simulink model "ISA"  (R2018b)
settings: Solver=FixedStepDiscrete  StartTime=0.0  StopTime=10  FixedStep=0.01  RelTol=1e-3
PreLoadFcn:
  | librarySetup
  | eval([bdroot,'_startup']) %Calling [modelName]_startup.m
values from neighbouring files (symbols this model uses):
  PWM_motor = 0.6    [ISA_simulation_startup.m]    (also in ISA_startup.m)
  V_max = 50    [ISA_startup.m]
libraries: HANcoder_STM32_Target x5, HANcoder_STM32_Target2009b x2, simulink x1
CloseFcn:
  | rtwprivate ssgencode ModelCloseRequest mytest
settings Model: Creator=Saliou  LastModifiedBy=Saliou
settings SolverCC: PositivePriorityOrder=on
settings DataIOCC: LimitDataPoints=on  SaveFormat=Array  SaveOutput=off  SaveTime=off
settings OptimizationCC: BlockReduction=off  DefaultParameterBehavior=Inlined  DefaultUnderspecifiedDataType=single  InlineInvariantSignals=on  ExpressionDepthLimit=2147483647  StateBitsets=on  DataBitsets=on  ZeroExternalMemoryAtStartup=off  ZeroInternalMemoryAtStartup=off  InitFltsAndDblsToZero=on  NoFixptDivByZeroProtection=on  EfficientFloat2IntCast=on  LifeSpan=inf
settings DebuggingCC: SaveWithDisabledLinksMsg=none  SaveWithParameterizedLinksMsg=none  CheckSSInitialOutputMsg=off  UnderspecifiedInitializationDetection=Classic  MergeDetectMultiDrivingBlocksExec=none  SignalResolutionControl=TryResolveAll  SolverPrmCheckMsg=warning  InheritedTsInSrcMsg=none  MultiTaskDSMMsg=warning  MultiTaskCondExecSysMsg=none  ParameterPrecisionLossMsg=none  FcnCallInpInsideContextMsg=warning  StateNameClashWarn=warning  SFUnexpectedBacktrackingDiag=warning  SFNoUnconditionalDefaultTransitionDiag=warning  SFExecutionAtInitializationDiag=none
settings HardwareCC: ProdBitPerPointer=32  ProdBitPerSizeT=32  ProdBitPerPtrDiffT=32  ProdLargestAtomicInteger=Long  ProdLargestAtomicFloat=Double  ProdWordSize=32  ProdHWDeviceType=ARM Compatible->ARM Cortex  TargetEndianess=LittleEndian  TargetHWDeviceType=Infineon->TriCore
settings ModelReferenceCC: PropagateSignalLabelsOutOfModel=off
settings SFSimCC: SimUseLocalCustomCode=off  MATLABDynamicMemAlloc=off
settings RTWCC: SystemTargetFile=ert.tlc  MakeCommand=make_rtw SHELL= HANcoder_PORTABLE=1 HANcoder_BOOTLOADER=1  TemplateMakefile=Olimexino_STM32_gcc.tmf  Description=Real-Time Workshop Embedded Coder (no auto configuration)  RTWUseLocalCustomCode=off
settings CodeAppCC: ForceParamTrailComments=on  IgnoreCustomStorageClasses=off  SimulinkDataObjDesc=on  CustomSymbolStrGlobalVar=rt$N$M  CustomSymbolStrType=$N$M  CustomSymbolStrFcn=$N$M$F  CustomSymbolStrMacro=$N$M  InsertBlockDesc=on  StateflowObjectComments=on  InternalIdentifier=Classic
settings ERTTargetCC: TargetFcnLib=ansi_tfl_tmw.mat  MultiwordLength=2048  IncludeMdlTerminateFcn=off  SuppressErrorStatus=on  SupportNonFinite=off  GenerateASAP2=on  InlinedParameterPlacement=NonHierarchical  ERTCustomFileTemplate=example_file_process.tlc  ConvertIfToSwitch=off  SuppressUnreachableDefaultCases=off
settings ConfigComp: CovMetricSettings=dw  CovHtmlReporting=on  CovSaveCumulativeToWorkspaceVar=on  CovSaveSingleToWorkspaceVar=on  CovExternalEMLEnable=off  CovSFcnEnable=off  DVMaxProcessTime=600  DVDisplayUnsatisfiableObjectives=on  DVAutomaticStubbing=off  DVModelCoverageObjectives=MCDC  DVMaxTestCaseSteps=500  DVTestSuiteOptimization=CombinedObjectives  DVDetectActiveLogic=on  DVSaveHarnessModel=on

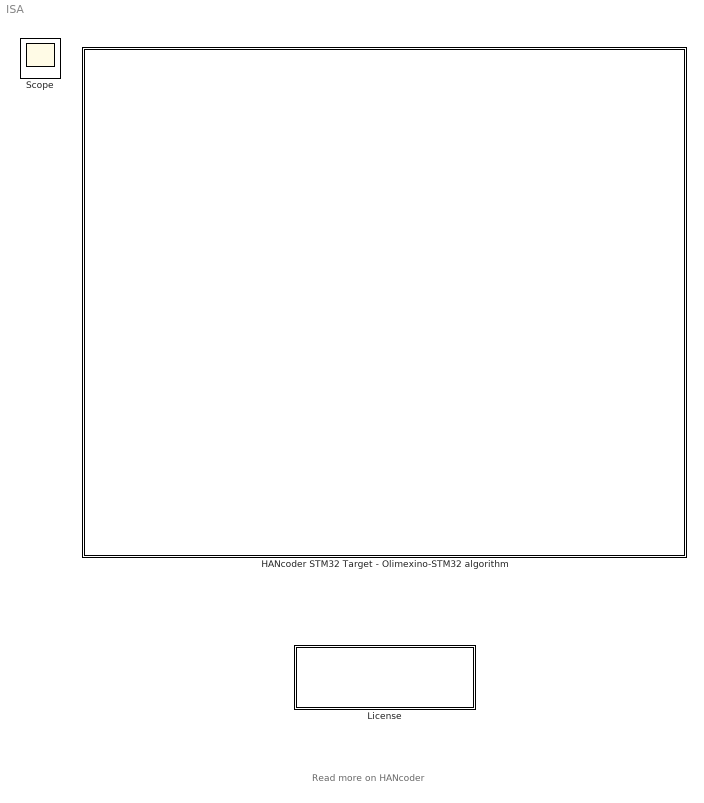
== system ISA ==
  note: Read more on HANcoder
  HANcoder STM32 Target - Olimexino-STM32 algorithm : Subsystem  mask(TopLevelSubsystem){}
      settings: CopyFcn=HANcoderChecks('Copy');  NameChangeFcn=HANcoderChecks('NameChangeOlimexino');  MoveFcn=HANcoderChecks('MoveOlimexino');
      mask Display: image(imread('Olimexino_STM32_HAN.jpg'))
  License : Subsystem  mask(License){}
      settings: NameChangeFcn=HANcoderChecks('NameChangeLicenseBlock');  OpenFcn=winopen('License.pdf')  MoveFcn=HANcoderChecks('MoveLicenseBlock');
      mask Display: disp(['End-User License Agreement\n','please read before use']);
  Scope : Scope

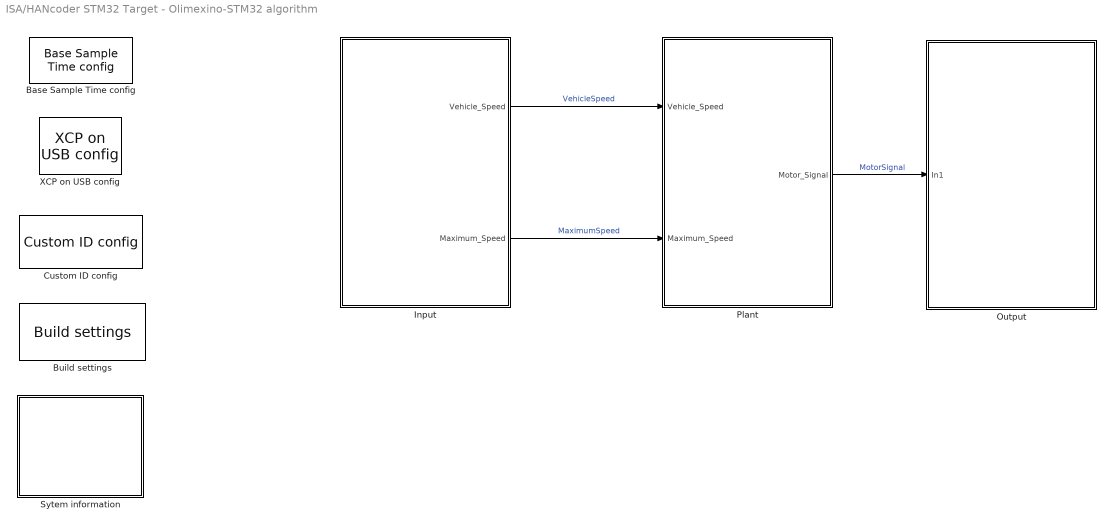
== system ISA/HANcoder STM32 Target - Olimexino-STM32 algorithm ==
  Base Sample Time config : HANcoder_STM32_Target/Olimexino STM32/System Config/Base Sample Time config  Tag=HANcoder_TARGET_STM32_Olimexino  Description=HANcoder Target STM32-Olimexino blockset version 1.0  baseSampleTime=10  extraStack=0
      settings: SourceProductName=HANcoder STM32 Target
  Build settings : HANcoder_STM32_Target/Olimexino STM32/System Config/Build settings  Tag=HANcoder_TARGET_STM32_Olimexino  AutoASAP2add=on  AutoFlash=USB
      settings: SourceProductName=HANcoder STM32 Target
  Custom ID config : HANcoder_STM32_Target2009b/Olimexino STM32/System Config/Custom ID config  Tag=HANcoder_TARGET_STM32_Olimexino  softID=softwareID  softNUM=1
  Input : Subsystem
  Output : Subsystem
  Plant : Subsystem
  Sytem information : Subsystem
  XCP on USB config : HANcoder_STM32_Target2009b/Olimexino STM32/System Config/XCP on USB config  Tag=HANcoder_TARGET_STM32_Olimexino
  wires:
  Plant/1(Motor_Signal) -> Output/1(In1)  "MotorSignal"
  Input/1(Vehicle_Speed) -> Plant/1(Vehicle_Speed)  "VehicleSpeed"
  Input/2(Maximum_Speed) -> Plant/2(Maximum_Speed)  "MaximumSpeed"

== system ISA/License ==

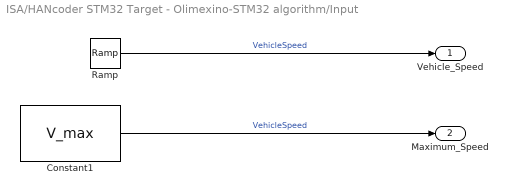
== system ISA/HANcoder STM32 Target - Olimexino-STM32 algorithm/Input ==
  Constant1 : Constant  Value=V_max  OutDataTypeStr=single
  Ramp : simulink/Sources/Ramp  slope=6  start=0  InitialOutput=0
  Vehicle_Speed : Outport
  Maximum_Speed : Outport  Port=2
  wires:
  Ramp/1 -> Vehicle_Speed/1  "VehicleSpeed"
  Constant1/1 -> Maximum_Speed/1  "VehicleSpeed"

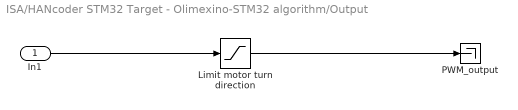
== system ISA/HANcoder STM32 Target - Olimexino-STM32 algorithm/Output ==
  In1 : Inport
  Limit motor turn direction : Saturate  UpperLimit=0.6  LowerLimit=0
  PWM_output : Terminator
  wires:
  In1/1 -> Limit motor turn direction/1
  Limit motor turn direction/1 -> PWM_output/1

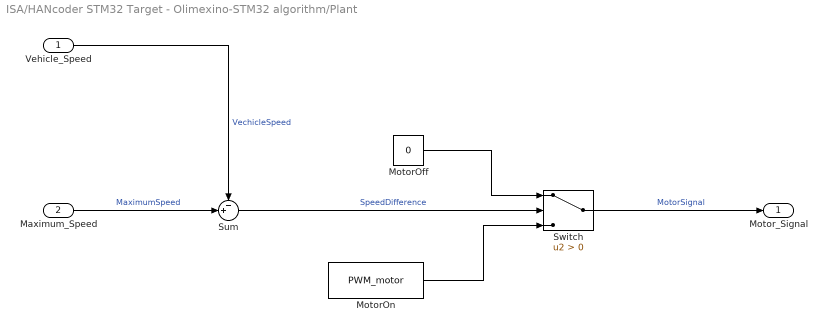
== system ISA/HANcoder STM32 Target - Olimexino-STM32 algorithm/Plant ==
  Vehicle_Speed : Inport
  Maximum_Speed : Inport  Port=2
  MotorOff : Constant  Value=0
  MotorOn : Constant  Value=PWM_motor
  Sum : Sum  Inputs=-+|
  Switch : Switch  Criteria=u2 > Threshold
  Motor_Signal : Outport
  wires:
  Maximum_Speed/1 -> Sum/2  "MaximumSpeed"
  Vehicle_Speed/1 -> Sum/1  "VechicleSpeed"
  Sum/1 -> Switch/2  "SpeedDifference"
  Switch/1 -> Motor_Signal/1  "MotorSignal"
  MotorOn/1 -> Switch/3
  MotorOff/1 -> Switch/1

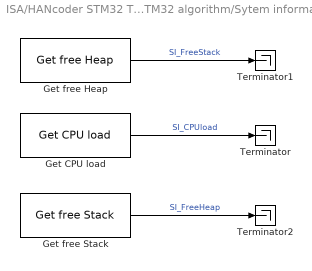
== system ISA/HANcoder STM32 Target - Olimexino-STM32 algorithm/Sytem information ==
  Get CPU load : HANcoder_STM32_Target/Olimexino STM32/System Management/Get CPU load  Tag=HANcoder_TARGET_STM32_Olimexino  mode=Current CPU load  tsamp=-1
      settings: SourceProductName=HANcoder STM32 Target
  Get free Heap : HANcoder_STM32_Target/Olimexino STM32/System Management/Get free Heap  Tag=HANcoder_TARGET_STM32_Olimexino  tsamp=-1
      settings: SourceProductName=HANcoder STM32 Target
  Get free Stack : HANcoder_STM32_Target/Olimexino STM32/System Management/Get free Stack  Tag=HANcoder_TARGET_STM32_Olimexino  taskIdx=Application Control Task  tsamp=-1
      settings: SourceProductName=HANcoder STM32 Target
  Terminator : Terminator
  Terminator1 : Terminator
  Terminator2 : Terminator
  wires:
  Get CPU load/1 -> Terminator/1  "SI_CPUload"
  Get free Heap/1 -> Terminator1/1  "SI_FreeStack"
  Get free Stack/1 -> Terminator2/1  "SI_FreeHeap"
